simulink model "simulink_continu_p1"  (Simulink 8.4)
settings: Solver=ode45  StartTime=0.0  StopTime=10.0  RelTol=1e-3
values from neighbouring files (symbols this model uses):
  K = acker(A,B,[-5+20*i -5-20*i])    [doble_integrador.m]    (also in matlab.mat = [0.749701499402 -0.42000042])
settings Model: Creator=student  LastModifiedBy=lluis
settings DebuggingCC: FcnCallInpInsideContextMsg=EnableAllAsWarning

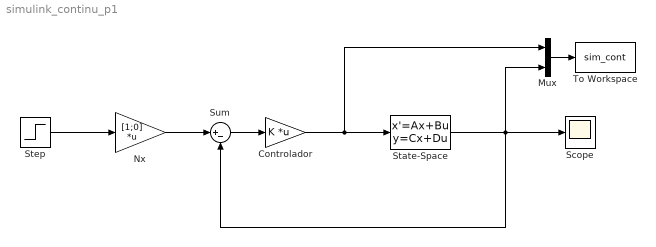
== system simulink_continu_p1 ==
  Controlador : Gain  Gain=K  Multiplication=Matrix(K*u)
  Mux : Mux  Inputs=2
  Nx : Gain  Gain=[1;0]  Multiplication=Matrix(K*u)
  Scope : Scope
  State-Space : StateSpace  A=[0 -23.8095;0 0]  B=[0;-23.8095]  C=[1 0;0 1]  D=[0; 0]  X0=1
  Step : Step  After=2  SampleTime=0
  Sum : Sum  Inputs=|+-
  To Workspace : ToWorkspace  VariableName=sim_cont  SaveFormat=Timeseries  SampleTime=-1
  wires:
  Sum/1 -> Controlador/1
  Step/1 -> Nx/1
  Nx/1 -> Sum/1
  Controlador/1 -> Mux/1, State-Space/1
  State-Space/1 -> Mux/2, Sum/2, Scope/1
  Mux/1 -> To Workspace/1
